simulink model "full_maneuver_platoon"  (R2022a)
settings: Solver=ode23t  StartTime=0.0  StopTime=300  FixedStep=0.1  MaxStep=0.01  RelTol=1e-3
InitFcn:
  | totalVehicles = 7;
  | if exist('vehStatesBus', 'var')==0
  | load vehBuses
  | end
  | if exist('vehErrorsBus', 'var')==0
  | load vehBuses
  | end
libraries: simulink x80, powerlib_meascontrol x16, autolibshared x7, dspsigops x4
(part 7 of 9)

== system full_maneuver_platoon/p1/CACC destination lane/Virtual Vehicle Following/Define Desired Distance ==
  extraSpaceFlag : Inport
  Constant : Constant  Value=h
  Constant1 : Constant  Value=d0
  Constant2 : Constant  Value=hLC
  Constant3 : Constant  Value=d0LC
  Demux : Demux  Outputs=2
  Integrator : Integrator  InitialCondition=[h d0]
  Mux : Mux  Inputs=2
  Mux1 : Mux  Inputs=2
  Saturation1 : Saturate  UpperLimit=hFilterSaturation/2  LowerLimit=-hFilterSaturation
  Sum5 : Sum  Inputs=|+-
  Switch : Switch  Criteria=u2 > Threshold  SaturateOnIntegerOverflow=off  InputSameDT=off
  hFilterGain : Gain  Gain=hFilterGain
  h : Outport
  d0 : Outport  Port=2
  wires:
  Demux/2 -> d0/1
  Demux/1 -> h/1
  Integrator/1 -> Sum5/2, Demux/1
  Saturation1/1 -> Integrator/1
  extraSpaceFlag/1 -> Switch/2
  Constant1/1 -> Mux/2
  Constant3/1 -> Mux1/2
  Switch/1 -> Sum5/1
  Mux1/1 -> Switch/1
  Sum5/1 -> hFilterGain/1
  Constant2/1 -> Mux1/1
  hFilterGain/1 -> Saturation1/1
  Constant/1 -> Mux/1
  Mux/1 -> Switch/3

== system full_maneuver_platoon/p1/CACC destination lane/Virtual Vehicle Following/Min Velocity Control ==
  ev : Inport
  ea : Inport  Port=2
  intergralReset : Inport  Port=3
  Abs : Abs  SaturateOnIntegerOverflow=off
  Compare To Constant : simulink/Logic and Bit Operations/Compare To Constant  relop=<=  const=2*maxComfAccel  OutDataTypeStr=boolean
  Gain : Gain  Gain=velKd
  Scope : Scope  NumInputPorts=4
  Sum3 : Sum  Inputs=+++
  Transport Delay : TransportDelay  DelayTime=0.1
  integral term : Subsystem
  velKp : Gain  Gain=velKp
  u : Outport  VectorParamsAs1DForOutWhenUnconnected=off
  wires:
  Compare To Constant/1 -> integral term/Enable
  integral term/1(Out1) -> Sum3/1, Scope/1
  Abs/1 -> Compare To Constant/1
  Transport Delay/1 -> Abs/1
  ev/1 -> velKp/1, integral term/1(ev)
  velKp/1 -> Scope/2, Sum3/2
  Sum3/1 -> u/1, Scope/4, Transport Delay/1
  intergralReset/1 -> integral term/2(intergralReset)
  ea/1 -> Gain/1
  Gain/1 -> Scope/3, Sum3/3

== system full_maneuver_platoon/p1/CACC destination lane/Virtual Vehicle Following/Velocity Error ==
  ego : Inport
  velRef : Inport  Port=2
  filterReset : Inport  Port=3
  Bus Selector : BusSelector  OutputSignals=Xdot,xddot
  Gain : Gain  Gain=-1
  Gain3 : Gain  Gain=velFilterGain
  Integrator1 : Integrator  ExternalReset=rising  InitialConditionSource=external  InitialCondition=vx0
  Saturation : Saturate  UpperLimit=maxComfAccel  LowerLimit=minComfAccel
  Sum : Sum  Inputs=+-|
  Sum8 : Sum  Inputs=|+-
  ev : Outport
  ea : Outport  Port=2
  wires:
  Sum8/1 -> Gain3/1
  Gain3/1 -> Saturation/1
  Saturation/1 -> Integrator1/1
  velRef/1 -> Sum8/1
  Integrator1/1 -> Sum/1, Sum8/2
  ego/1 -> Bus Selector/1
  Bus Selector/1 -> Sum/2, Integrator1/3  "<Xdot>"
  Bus Selector/2 -> Gain/1  "<xddot>"
  Sum/1 -> ev/1
  Gain/1 -> ea/1
  filterReset/1 -> Integrator1/2

== system full_maneuver_platoon/p1/CACC destination lane/Virtual Vehicle Following/Virtual Leader Following ==
  errors : Inport
  errorsDot : Inport  Port=2
  realInput : Inport  Port=3
  leaderChange : Inport  Port=4
  inRange : Inport  Port=5
  AND : Logic  IconShape=distinctive  AllPortsSameDT=off  OutDataTypeStr=boolean
  Compare To Constant : simulink/Logic and Bit Operations/Compare To Constant  relop=~=  const=0  OutDataTypeStr=boolean
  Constant : Constant  Value=Ki
  Demux : Demux  Outputs=2
  Demux1 : Demux  Outputs=2
  Gain3 : Gain  Gain=Ka
  Gain4 : Gain  Gain=Kdd
  Gain5 : Gain  Commented=on  Gain=10
  Integrator1 : Integrator  Commented=on  ExternalReset=rising  InitialConditionSource=external  InitialCondition=vx0
  Kd : Gain  Gain=Kd
  Kp : Gain  Gain=Kp
  Saturation : Saturate  Commented=on  UpperLimit=maxComfAccel  LowerLimit=minAcceleration
  Saturation1 : Saturate  UpperLimit=maxGapError  LowerLimit=minGapError
  Scope : Scope  NumInputPorts=6
  Sum : Sum  Inputs=+-|
  Sum1 : Sum  Inputs=+++++
  Sum8 : Sum  Commented=on  Inputs=|+-
  Transport Delay : TransportDelay  DelayTime=0.1
  integralTerm : Subsystem
  u : Outport  VectorParamsAs1DForOutWhenUnconnected=off
  wires:
  errorsDot/1 -> Demux1/1
  errors/1 -> Demux/1
  Demux/1 -> Saturation1/1
  Kd/1 -> Scope/3, Sum1/3
  Gain5/1 -> Saturation/1
  inRange/1 -> AND/2, Integrator1/2
  Transport Delay/1 -> Scope/1, Sum1/1
  Saturation1/1 -> integralTerm/1(eh), Kp/1
  Kp/1 -> Scope/2, Sum1/2
  Sum/1 -> integralTerm/2(inputDiff)
  Sum8/1 -> Gain5/1
  realInput/1 -> Integrator1/3, Sum/2
  Gain4/1 -> Scope/4, Sum1/4
  Saturation/1 -> Integrator1/1
  Demux/2 -> Kd/1  "ev"
  Gain3/1 -> Scope/5, Sum1/5
  Integrator1/1 -> Sum8/2
  Sum1/1 -> u/1, Scope/6, Sum/1
  integralTerm/1(Out1) -> Transport Delay/1
  leaderChange/1 -> integralTerm/3(leaderChange)
  Demux1/1 -> Gain4/1  "egDot"
  Demux1/2 -> Gain3/1  "evDot"
  Constant/1 -> Compare To Constant/1
  Compare To Constant/1 -> AND/1
  AND/1 -> integralTerm/Enable

== system full_maneuver_platoon/p1/CACC destination lane/Virtual Vehicle Following/switch min vel ==
  errors : Inport
  errorsDot : Inport  Port=2
  gap : Inport  Port=3
  h : Inport  Port=4
  d0 : Inport  Port=5
  vRef : Inport  Port=6
  Demux1 : Demux  Outputs=2
  Gain1 : Gain
  MATLAB Function : MATLAB Function  TreatAsAtomicUnit=on
  Relay1 : Relay  OnSwitchValue=1  OffSwitchValue=-1
  Scope : Scope  NumInputPorts=2
  Selector : Selector  InputPortWidth=2  IndexOptions=Index vector (dialog)  Indices=[2]  OutputSizes=1
  Sum2 : Sum  Inputs=-+
  inRange : Outport  VectorParamsAs1DForOutWhenUnconnected=off
  wires:
  Demux1/2 -> MATLAB Function/6(ea)
  Demux1/1 -> MATLAB Function/5(ehDot)
  errorsDot/1 -> Demux1/1
  MATLAB Function/1(maxGap) -> Sum2/2, Scope/2
  Gain1/1 -> MATLAB Function/1(h)
  Relay1/1 -> inRange/1
  Selector/1 -> MATLAB Function/4(ev)
  Sum2/1 -> Relay1/1
  gap/1 -> Sum2/1, Scope/1
  errors/1 -> Selector/1
  h/1 -> Gain1/1
  vRef/1 -> MATLAB Function/3(vRef)
  d0/1 -> MATLAB Function/2(d0)

== system full_maneuver_platoon/p1/CACC origin lane/Veh Following/integralTerm ==
  eh : Inport
  inputDiff : Inport  Port=2
  leaderChange : Inport  Port=3
  Enable : EnablePort  ShowOutputPort=on
  Anti-windup gain : Gain  Gain=sqrt(Ki/Kd)
  Integrator : Integrator  ExternalReset=either
  Ki : Gain  Gain=Ki
  Scope : Scope  NumInputPorts=2
  Sum5 : Sum  Inputs=-+|
  XOR : Logic  Operator=XOR  IconShape=distinctive  AllPortsSameDT=off  OutDataTypeStr=boolean
  Out1 : Outport  OutputWhenDisabled=reset  InitialOutput=0  VectorParamsAs1DForOutWhenUnconnected=off
  wires:
  inputDiff/1 -> Anti-windup gain/1
  Anti-windup gain/1 -> Scope/1, Sum5/1
  Ki/1 -> Sum5/2
  Sum5/1 -> Scope/2, Integrator/1
  Enable/1 -> XOR/2
  leaderChange/1 -> XOR/1
  XOR/1 -> Integrator/2
  Integrator/1 -> Out1/1
  eh/1 -> Ki/1

== system full_maneuver_platoon/p1/CACC origin lane/Velocity Control/integral term ==
  ev : Inport
  integralReset : Inport  Port=2
  Enable : EnablePort  StatesWhenEnabling=reset
  Integrator2 : Integrator  ExternalReset=rising
  velKi : Gain  Gain=velKi
  Out1 : Outport  OutputWhenDisabled=reset  InitialOutput=0
  wires:
  ev/1 -> velKi/1
  Integrator2/1 -> Out1/1
  velKi/1 -> Integrator2/1
  integralReset/1 -> Integrator2/2

== system full_maneuver_platoon/p1/Lane Change Strategy/Strategy 1: synchronous/determine virtual follower idx ==
  note: In the synchronous strategy, only the last platoon vehicles has a virtual follower,
      | which is the follower in the destination lane (fd) as virtual follower. The index of
      | fd in the allVehicles array is 2
  Enable : EnablePort
  Constant : Constant  Value=2
  virtualFollowerIdx : Outport  OutputWhenDisabled=reset  InitialOutput=[0]
  wires:
  Constant/1 -> virtualFollowerIdx/1

== system full_maneuver_platoon/p1/Lane Change Strategy/Strategy 1: synchronous/determine virtual leader idx ==
  nVehicles : Inport
  lcFlag : Inport  Port=2
  Enable : EnablePort
  determineVirtualLeader : MATLAB Function  TreatAsAtomicUnit=on
  virtualLeaderIdx : Outport  InitialOutput=0
  wires:
  lcFlag/1 -> determineVirtualLeader/2(lcFlag)
  determineVirtualLeader/1(virtualLeaderIdx) -> virtualLeaderIdx/1
  nVehicles/1 -> determineVirtualLeader/1(nVehicles)

== system full_maneuver_platoon/p1/Lane Change Strategy/Strategy 2: leader first/determine virtual follower idx ==
  note: In the leader first strategy, all vehicles have the follower in the destination lane (fd)
      | as virtual follower. The index of fd in the allVehicles array is 2
  Enable : EnablePort
  Constant : Constant  Value=2
  virtualFollowerIdx : Outport  OutputWhenDisabled=reset  InitialOutput=[0]
  wires:
  Constant/1 -> virtualFollowerIdx/1

== system full_maneuver_platoon/p1/Lane Change Strategy/Strategy 2: leader first/determine virtual leader idx ==
  nVehicles : Inport
  lcFlag : Inport  Port=2
  posInPlatoon : Inport  Port=3
  Enable : EnablePort
  determineVirtualLeader : MATLAB Function  TreatAsAtomicUnit=on
  virtualLeaderIdx : Outport  InitialOutput=[0]
  wires:
  posInPlatoon/1 -> determineVirtualLeader/3(posInPlatoon)
  determineVirtualLeader/1(virtualLeaderIdx) -> virtualLeaderIdx/1  "virtualLeaderIdx"
  lcFlag/1 -> determineVirtualLeader/2(lcFlag)
  nVehicles/1 -> determineVirtualLeader/1(nVehicles)

== system full_maneuver_platoon/p1/Lane Change Strategy/Strategy 3: last first/determine virtual follower idx ==
  platoonSize : Inport
  posInPlatoon : Inport  Port=2
  Enable : EnablePort
  determineVirtualFollower : MATLAB Function  TreatAsAtomicUnit=on
  virtual follower idx : Outport  OutputWhenDisabled=reset  InitialOutput=[0]
  wires:
  posInPlatoon/1 -> determineVirtualFollower/2(posInPlatoon)
  determineVirtualFollower/1(virtualFollowerIdx) -> virtual follower idx/1
  platoonSize/1 -> determineVirtualFollower/1(platoonSize)

== system full_maneuver_platoon/p1/Lane Change Strategy/Strategy 3: last first/determine virtual leader idx ==
  nVehicles : Inport
  lcFlag : Inport  Port=2
  lcDone : Inport  Port=3
  posInPlatoon : Inport  Port=4
  Enable : EnablePort
  determineVirtualLeader : MATLAB Function  TreatAsAtomicUnit=on
  virtualLeaderIdx : Outport  InitialOutput=[0]
  wires:
  nVehicles/1 -> determineVirtualLeader/1(nVehicles)
  posInPlatoon/1 -> determineVirtualLeader/4(posInPlatoon)
  lcFlag/1 -> determineVirtualLeader/2(lcFlag)
  lcDone/1 -> determineVirtualLeader/3(lcDone)
  determineVirtualLeader/1(virtualLeaderIdx) -> virtualLeaderIdx/1

== system full_maneuver_platoon/p1/Lane Change Strategy/Strategy 4: leader first invert/Subsystem ==
  posInPlatoon : Inport
  Enable : EnablePort
  determineVirtualFollower : MATLAB Function  TreatAsAtomicUnit=on
  virtualFollowerIdx : Outport  OutputWhenDisabled=reset  InitialOutput=[0]
  wires:
  determineVirtualFollower/1(virtualFollowerIdx) -> virtualFollowerIdx/1
  posInPlatoon/1 -> determineVirtualFollower/1(posInPlatoon)

== system full_maneuver_platoon/p1/Lane Change Strategy/Strategy 4: leader first invert/Subsystem1 ==
  nVehicles : Inport
  lcFlag : Inport  Port=2
  lcDone : Inport  Port=3
  posInPlatoon : Inport  Port=4
  Enable : EnablePort
  determineVirtualLeader : MATLAB Function  TreatAsAtomicUnit=on
  virtualLeaderIdx : Outport  InitialOutput=[0]
  wires:
  lcDone/1 -> determineVirtualLeader/3(lcDone)
  nVehicles/1 -> determineVirtualLeader/1(nVehicles)
  lcFlag/1 -> determineVirtualLeader/2(lcFlag)
  posInPlatoon/1 -> determineVirtualLeader/4(posInPlatoon)
  determineVirtualLeader/1(virtualLeaderIdx) -> virtualLeaderIdx/1

== system full_maneuver_platoon/p2/CACC destination lane/Virtual Vehicle Following/Compute Errors ==
  ego : Inport
  leader : Inport  Port=2
  h : Inport  Port=3
  d0 : Inport  Port=4
  velFilterReset : Inport  Port=5
  Bus Selector1 : BusSelector  OutputSignals=X,Xdot,xddot
  Bus Selector2 : BusSelector  OutputSignals=X,Xdot,xddot
  Compare To Constant : simulink/Logic and Bit Operations/Compare To Constant  relop=<  const=0  OutDataTypeStr=boolean
  Gain3 : Gain  Gain=velFilterGain
  Integrator1 : Integrator  ExternalReset=rising  InitialCondition=vx0
  Multiply : Product
  Multiply1 : Product
  Mux2 : Mux  Inputs=2
  Mux3 : Mux  Inputs=2
  Product : Product
  Saturation : Saturate  UpperLimit=maxAcceleration  LowerLimit=minAcceleration
  Sum : Sum  Inputs=|-+
  Sum1 : Sum  Inputs=|++
  Sum10 : Sum  Inputs=+-|
  Sum2 : Sum  Inputs=+-|
  Sum3 : Sum  Inputs=|++
  Sum4 : Sum  Inputs=-+|
  Sum6 : Sum  Inputs=|-+
  Sum7 : Sum  Inputs=++|
  Sum8 : Sum  Inputs=|+-
  Sum9 : Sum  Inputs=-+|
  min d0 : Constant  Value=d0
  min h : Constant  Value=h
  vLen : Constant  Value=lr+lf
  errors : Outport  VectorParamsAs1DForOutWhenUnconnected=off
  errorsDot : Outport  Port=2
  "gap " : Outport  Port=3  VectorParamsAs1DForOutWhenUnconnected=off
  unsafeFlag : Outport  Port=4  VectorParamsAs1DForOutWhenUnconnected=off
  wires:
  Mux2/1 -> errors/1
  velFilterReset/1 -> Integrator1/2
  Sum6/1 -> Compare To Constant/1
  Sum7/1 -> Sum6/1  "safe  gap"
  min h/1 -> Product/1
  Compare To Constant/1 -> unsafeFlag/1
  Sum2/1 -> Mux2/1  "eg"
  Bus Selector1/1 -> Sum/2  "<X>"
  Product/1 -> Sum7/2
  Sum3/1 -> Sum2/2  "desired  gap"
  Sum1/1 -> Sum/1  "x (front bumber)"
  Bus Selector2/2 -> Sum4/1, Multiply/1, Product/2  "<Xdot>"
  d0/1 -> Sum3/2
  vLen/1 -> Sum1/1
  min d0/1 -> Sum7/1
  Multiply/1 -> Sum3/1
  Sum/1 -> Sum2/1, "gap "/1, Sum6/2  "gap"
  Bus Selector2/1 -> Sum1/2  "<X>"
  h/1 -> Multiply/2, Multiply1/1
  Bus Selector1/2 -> Sum8/1  "<Xdot>"
  Sum4/1 -> Mux2/2, Sum10/1  "ev"
  Gain3/1 -> Saturation/1
  Saturation/1 -> Integrator1/1
  Integrator1/1 -> Sum4/2, Sum8/2
  Sum8/1 -> Gain3/1
  Bus Selector1/3 -> Sum9/2  "<xddot>"
  Bus Selector2/3 -> Sum9/1, Multiply1/2  "<xddot>"
  Multiply1/1 -> Sum10/2
  Sum10/1 -> Mux3/1  "egDot"
  Sum9/1 -> Mux3/2  "evDot"
  Mux3/1 -> errorsDot/1
  ego/1 -> Bus Selector2/1
  leader/1 -> Bus Selector1/1

== system full_maneuver_platoon/p2/CACC destination lane/Virtual Vehicle Following/Define Desired Distance ==
  extraSpaceFlag : Inport
  Constant : Constant  Value=h
  Constant1 : Constant  Value=d0
  Constant2 : Constant  Value=hLC
  Constant3 : Constant  Value=d0LC
  Demux : Demux  Outputs=2
  Integrator : Integrator  InitialCondition=[h d0]
  Mux : Mux  Inputs=2
  Mux1 : Mux  Inputs=2
  Saturation1 : Saturate  UpperLimit=hFilterSaturation/2  LowerLimit=-hFilterSaturation
  Sum5 : Sum  Inputs=|+-
  Switch : Switch  Criteria=u2 > Threshold  SaturateOnIntegerOverflow=off  InputSameDT=off
  hFilterGain : Gain  Gain=hFilterGain
  h : Outport
  d0 : Outport  Port=2
  wires:
  Mux/1 -> Switch/3
  Constant/1 -> Mux/1
  hFilterGain/1 -> Saturation1/1
  Constant2/1 -> Mux1/1
  Sum5/1 -> hFilterGain/1
  Mux1/1 -> Switch/1
  Switch/1 -> Sum5/1
  Constant3/1 -> Mux1/2
  Constant1/1 -> Mux/2
  extraSpaceFlag/1 -> Switch/2
  Saturation1/1 -> Integrator/1
  Integrator/1 -> Demux/1, Sum5/2
  Demux/1 -> h/1
  Demux/2 -> d0/1

== system full_maneuver_platoon/p2/CACC destination lane/Virtual Vehicle Following/Min Velocity Control ==
  ev : Inport
  ea : Inport  Port=2
  intergralReset : Inport  Port=3
  Abs : Abs  SaturateOnIntegerOverflow=off
  Compare To Constant : simulink/Logic and Bit Operations/Compare To Constant  relop=<=  const=2*maxComfAccel  OutDataTypeStr=boolean
  Gain : Gain  Gain=velKd
  Scope : Scope  NumInputPorts=4
  Sum3 : Sum  Inputs=+++
  Transport Delay : TransportDelay  DelayTime=0.1
  integral term : Subsystem
  velKp : Gain  Gain=velKp
  u : Outport  VectorParamsAs1DForOutWhenUnconnected=off
  wires:
  Gain/1 -> Sum3/3, Scope/3
  ea/1 -> Gain/1
  intergralReset/1 -> integral term/2(intergralReset)
  Sum3/1 -> Transport Delay/1, Scope/4, u/1
  velKp/1 -> Sum3/2, Scope/2
  ev/1 -> integral term/1(ev), velKp/1
  Transport Delay/1 -> Abs/1
  Abs/1 -> Compare To Constant/1
  integral term/1(Out1) -> Scope/1, Sum3/1
  Compare To Constant/1 -> integral term/Enable

== system full_maneuver_platoon/p2/CACC destination lane/Virtual Vehicle Following/Velocity Error ==
  ego : Inport
  velRef : Inport  Port=2
  filterReset : Inport  Port=3
  Bus Selector : BusSelector  OutputSignals=Xdot,xddot
  Gain : Gain  Gain=-1
  Gain3 : Gain  Gain=velFilterGain
  Integrator1 : Integrator  ExternalReset=rising  InitialConditionSource=external  InitialCondition=vx0
  Saturation : Saturate  UpperLimit=maxComfAccel  LowerLimit=minComfAccel
  Sum : Sum  Inputs=+-|
  Sum8 : Sum  Inputs=|+-
  ev : Outport
  ea : Outport  Port=2
  wires:
  filterReset/1 -> Integrator1/2
  Gain/1 -> ea/1
  Sum/1 -> ev/1
  Bus Selector/2 -> Gain/1  "<xddot>"
  Bus Selector/1 -> Integrator1/3, Sum/2  "<Xdot>"
  ego/1 -> Bus Selector/1
  Integrator1/1 -> Sum8/2, Sum/1
  velRef/1 -> Sum8/1
  Saturation/1 -> Integrator1/1
  Gain3/1 -> Saturation/1
  Sum8/1 -> Gain3/1

== system full_maneuver_platoon/p2/CACC destination lane/Virtual Vehicle Following/Virtual Leader Following ==
  errors : Inport
  errorsDot : Inport  Port=2
  realInput : Inport  Port=3
  leaderChange : Inport  Port=4
  inRange : Inport  Port=5
  AND : Logic  IconShape=distinctive  AllPortsSameDT=off  OutDataTypeStr=boolean
  Compare To Constant : simulink/Logic and Bit Operations/Compare To Constant  relop=~=  const=0  OutDataTypeStr=boolean
  Constant : Constant  Value=Ki
  Demux : Demux  Outputs=2
  Demux1 : Demux  Outputs=2
  Gain3 : Gain  Gain=Ka
  Gain4 : Gain  Gain=Kdd
  Gain5 : Gain  Commented=on  Gain=10
  Integrator1 : Integrator  Commented=on  ExternalReset=rising  InitialConditionSource=external  InitialCondition=vx0
  Kd : Gain  Gain=Kd
  Kp : Gain  Gain=Kp
  Saturation : Saturate  Commented=on  UpperLimit=maxComfAccel  LowerLimit=minAcceleration
  Saturation1 : Saturate  UpperLimit=maxGapError  LowerLimit=minGapError
  Scope : Scope  NumInputPorts=6
  Sum : Sum  Inputs=+-|
  Sum1 : Sum  Inputs=+++++
  Sum8 : Sum  Commented=on  Inputs=|+-
  Transport Delay : TransportDelay  DelayTime=0.1
  integralTerm : Subsystem
  u : Outport  VectorParamsAs1DForOutWhenUnconnected=off
  wires:
  AND/1 -> integralTerm/Enable
  Compare To Constant/1 -> AND/1
  Constant/1 -> Compare To Constant/1
  Demux1/2 -> Gain3/1  "evDot"
  Demux1/1 -> Gain4/1  "egDot"
  leaderChange/1 -> integralTerm/3(leaderChange)
  integralTerm/1(Out1) -> Transport Delay/1
  Sum1/1 -> Sum/1, Scope/6, u/1
  Integrator1/1 -> Sum8/2
  Gain3/1 -> Sum1/5, Scope/5
  Demux/2 -> Kd/1  "ev"
  Saturation/1 -> Integrator1/1
  Gain4/1 -> Sum1/4, Scope/4
  realInput/1 -> Sum/2, Integrator1/3
  Sum8/1 -> Gain5/1
  Sum/1 -> integralTerm/2(inputDiff)
  Kp/1 -> Sum1/2, Scope/2
  Saturation1/1 -> Kp/1, integralTerm/1(eh)
  Transport Delay/1 -> Sum1/1, Scope/1
  inRange/1 -> Integrator1/2, AND/2
  Gain5/1 -> Saturation/1
  Kd/1 -> Sum1/3, Scope/3
  Demux/1 -> Saturation1/1
  errors/1 -> Demux/1
  errorsDot/1 -> Demux1/1

== system full_maneuver_platoon/p2/CACC destination lane/Virtual Vehicle Following/switch min vel ==
  errors : Inport
  errorsDot : Inport  Port=2
  gap : Inport  Port=3
  h : Inport  Port=4
  d0 : Inport  Port=5
  vRef : Inport  Port=6
  Demux1 : Demux  Outputs=2
  Gain1 : Gain
  MATLAB Function : MATLAB Function  TreatAsAtomicUnit=on
  Relay1 : Relay  OnSwitchValue=1  OffSwitchValue=-1
  Scope : Scope  NumInputPorts=2
  Selector : Selector  InputPortWidth=2  IndexOptions=Index vector (dialog)  Indices=[2]  OutputSizes=1
  Sum2 : Sum  Inputs=-+
  inRange : Outport  VectorParamsAs1DForOutWhenUnconnected=off
  wires:
  d0/1 -> MATLAB Function/2(d0)
  vRef/1 -> MATLAB Function/3(vRef)
  h/1 -> Gain1/1
  errors/1 -> Selector/1
  gap/1 -> Scope/1, Sum2/1
  Sum2/1 -> Relay1/1
  Selector/1 -> MATLAB Function/4(ev)
  Relay1/1 -> inRange/1
  Gain1/1 -> MATLAB Function/1(h)
  MATLAB Function/1(maxGap) -> Scope/2, Sum2/2
  errorsDot/1 -> Demux1/1
  Demux1/1 -> MATLAB Function/5(ehDot)
  Demux1/2 -> MATLAB Function/6(ea)

== system full_maneuver_platoon/p2/CACC origin lane/Veh Following/integralTerm ==
  eh : Inport
  inputDiff : Inport  Port=2
  leaderChange : Inport  Port=3
  Enable : EnablePort  ShowOutputPort=on
  Anti-windup gain : Gain  Gain=sqrt(Ki/Kd)
  Integrator : Integrator  ExternalReset=either
  Ki : Gain  Gain=Ki
  Scope : Scope  NumInputPorts=2
  Sum5 : Sum  Inputs=-+|
  XOR : Logic  Operator=XOR  IconShape=distinctive  AllPortsSameDT=off  OutDataTypeStr=boolean
  Out1 : Outport  OutputWhenDisabled=reset  InitialOutput=0  VectorParamsAs1DForOutWhenUnconnected=off
  wires:
  eh/1 -> Ki/1
  Integrator/1 -> Out1/1
  XOR/1 -> Integrator/2
  leaderChange/1 -> XOR/1
  Enable/1 -> XOR/2
  Sum5/1 -> Integrator/1, Scope/2
  Ki/1 -> Sum5/2
  Anti-windup gain/1 -> Sum5/1, Scope/1
  inputDiff/1 -> Anti-windup gain/1

== system full_maneuver_platoon/p2/CACC origin lane/Velocity Control/integral term ==
  ev : Inport
  integralReset : Inport  Port=2
  Enable : EnablePort  StatesWhenEnabling=reset
  Integrator2 : Integrator  ExternalReset=rising
  velKi : Gain  Gain=velKi
  Out1 : Outport  OutputWhenDisabled=reset  InitialOutput=0
  wires:
  integralReset/1 -> Integrator2/2
  velKi/1 -> Integrator2/1
  Integrator2/1 -> Out1/1
  ev/1 -> velKi/1

== system full_maneuver_platoon/p2/Lane Change Strategy/Strategy 1: synchronous/determine virtual follower idx ==
  note: In the synchronous strategy, only the last platoon vehicles has a virtual follower,
      | which is the follower in the destination lane (fd) as virtual follower. The index of
      | fd in the allVehicles array is 2
  Enable : EnablePort
  Constant : Constant  Value=2
  virtualFollowerIdx : Outport  OutputWhenDisabled=reset  InitialOutput=[0]
  wires:
  Constant/1 -> virtualFollowerIdx/1

== system full_maneuver_platoon/p2/Lane Change Strategy/Strategy 1: synchronous/determine virtual leader idx ==
  nVehicles : Inport
  lcFlag : Inport  Port=2
  Enable : EnablePort
  determineVirtualLeader : MATLAB Function  TreatAsAtomicUnit=on
  virtualLeaderIdx : Outport  InitialOutput=0
  wires:
  nVehicles/1 -> determineVirtualLeader/1(nVehicles)
  determineVirtualLeader/1(virtualLeaderIdx) -> virtualLeaderIdx/1
  lcFlag/1 -> determineVirtualLeader/2(lcFlag)

== system full_maneuver_platoon/p2/Lane Change Strategy/Strategy 2: leader first/determine virtual follower idx ==
  note: In the leader first strategy, all vehicles have the follower in the destination lane (fd)
      | as virtual follower. The index of fd in the allVehicles array is 2
  Enable : EnablePort
  Constant : Constant  Value=2
  virtualFollowerIdx : Outport  OutputWhenDisabled=reset  InitialOutput=[0]
  wires:
  Constant/1 -> virtualFollowerIdx/1

== system full_maneuver_platoon/p2/Lane Change Strategy/Strategy 2: leader first/determine virtual leader idx ==
  nVehicles : Inport
  lcFlag : Inport  Port=2
  posInPlatoon : Inport  Port=3
  Enable : EnablePort
  determineVirtualLeader : MATLAB Function  TreatAsAtomicUnit=on
  virtualLeaderIdx : Outport  InitialOutput=[0]
  wires:
  nVehicles/1 -> determineVirtualLeader/1(nVehicles)
  lcFlag/1 -> determineVirtualLeader/2(lcFlag)
  determineVirtualLeader/1(virtualLeaderIdx) -> virtualLeaderIdx/1  "virtualLeaderIdx"
  posInPlatoon/1 -> determineVirtualLeader/3(posInPlatoon)

== system full_maneuver_platoon/p2/Lane Change Strategy/Strategy 3: last first/determine virtual follower idx ==
  platoonSize : Inport
  posInPlatoon : Inport  Port=2
  Enable : EnablePort
  determineVirtualFollower : MATLAB Function  TreatAsAtomicUnit=on
  virtual follower idx : Outport  OutputWhenDisabled=reset  InitialOutput=[0]
  wires:
  platoonSize/1 -> determineVirtualFollower/1(platoonSize)
  determineVirtualFollower/1(virtualFollowerIdx) -> virtual follower idx/1
  posInPlatoon/1 -> determineVirtualFollower/2(posInPlatoon)

== system full_maneuver_platoon/p2/Lane Change Strategy/Strategy 3: last first/determine virtual leader idx ==
  nVehicles : Inport
  lcFlag : Inport  Port=2
  lcDone : Inport  Port=3
  posInPlatoon : Inport  Port=4
  Enable : EnablePort
  determineVirtualLeader : MATLAB Function  TreatAsAtomicUnit=on
  virtualLeaderIdx : Outport  InitialOutput=[0]
  wires:
  determineVirtualLeader/1(virtualLeaderIdx) -> virtualLeaderIdx/1
  lcDone/1 -> determineVirtualLeader/3(lcDone)
  lcFlag/1 -> determineVirtualLeader/2(lcFlag)
  posInPlatoon/1 -> determineVirtualLeader/4(posInPlatoon)
  nVehicles/1 -> determineVirtualLeader/1(nVehicles)

== system full_maneuver_platoon/p2/Lane Change Strategy/Strategy 4: leader first invert/Subsystem ==
  posInPlatoon : Inport
  Enable : EnablePort
  determineVirtualFollower : MATLAB Function  TreatAsAtomicUnit=on
  virtualFollowerIdx : Outport  OutputWhenDisabled=reset  InitialOutput=[0]
  wires:
  posInPlatoon/1 -> determineVirtualFollower/1(posInPlatoon)
  determineVirtualFollower/1(virtualFollowerIdx) -> virtualFollowerIdx/1

== system full_maneuver_platoon/p2/Lane Change Strategy/Strategy 4: leader first invert/Subsystem1 ==
  nVehicles : Inport
  lcFlag : Inport  Port=2
  lcDone : Inport  Port=3
  posInPlatoon : Inport  Port=4
  Enable : EnablePort
  determineVirtualLeader : MATLAB Function  TreatAsAtomicUnit=on
  virtualLeaderIdx : Outport  InitialOutput=[0]
  wires:
  determineVirtualLeader/1(virtualLeaderIdx) -> virtualLeaderIdx/1
  posInPlatoon/1 -> determineVirtualLeader/4(posInPlatoon)
  lcFlag/1 -> determineVirtualLeader/2(lcFlag)
  nVehicles/1 -> determineVirtualLeader/1(nVehicles)
  lcDone/1 -> determineVirtualLeader/3(lcDone)

== system full_maneuver_platoon/p3/CACC destination lane/Virtual Vehicle Following/Compute Errors ==
  ego : Inport
  leader : Inport  Port=2
  h : Inport  Port=3
  d0 : Inport  Port=4
  velFilterReset : Inport  Port=5
  Bus Selector1 : BusSelector  OutputSignals=X,Xdot,xddot
  Bus Selector2 : BusSelector  OutputSignals=X,Xdot,xddot
  Compare To Constant : simulink/Logic and Bit Operations/Compare To Constant  relop=<  const=0  OutDataTypeStr=boolean
  Gain3 : Gain  Gain=velFilterGain
  Integrator1 : Integrator  ExternalReset=rising  InitialCondition=vx0
  Multiply : Product
  Multiply1 : Product
  Mux2 : Mux  Inputs=2
  Mux3 : Mux  Inputs=2
  Product : Product
  Saturation : Saturate  UpperLimit=maxAcceleration  LowerLimit=minAcceleration
  Sum : Sum  Inputs=|-+
  Sum1 : Sum  Inputs=|++
  Sum10 : Sum  Inputs=+-|
  Sum2 : Sum  Inputs=+-|
  Sum3 : Sum  Inputs=|++
  Sum4 : Sum  Inputs=-+|
  Sum6 : Sum  Inputs=|-+
  Sum7 : Sum  Inputs=++|
  Sum8 : Sum  Inputs=|+-
  Sum9 : Sum  Inputs=-+|
  min d0 : Constant  Value=d0
  min h : Constant  Value=h
  vLen : Constant  Value=lr+lf
  errors : Outport  VectorParamsAs1DForOutWhenUnconnected=off
  errorsDot : Outport  Port=2
  "gap " : Outport  Port=3  VectorParamsAs1DForOutWhenUnconnected=off
  unsafeFlag : Outport  Port=4  VectorParamsAs1DForOutWhenUnconnected=off
  wires:
  leader/1 -> Bus Selector1/1
  ego/1 -> Bus Selector2/1
  Mux3/1 -> errorsDot/1
  Sum9/1 -> Mux3/2  "evDot"
  Sum10/1 -> Mux3/1  "egDot"
  Multiply1/1 -> Sum10/2
  Bus Selector2/3 -> Multiply1/2, Sum9/1  "<xddot>"
  Bus Selector1/3 -> Sum9/2  "<xddot>"
  Sum8/1 -> Gain3/1
  Integrator1/1 -> Sum8/2, Sum4/2
  Saturation/1 -> Integrator1/1
  Gain3/1 -> Saturation/1
  Sum4/1 -> Sum10/1, Mux2/2  "ev"
  Bus Selector1/2 -> Sum8/1  "<Xdot>"
  h/1 -> Multiply1/1, Multiply/2
  Bus Selector2/1 -> Sum1/2  "<X>"
  Sum/1 -> Sum6/2, "gap "/1, Sum2/1  "gap"
  Multiply/1 -> Sum3/1
  min d0/1 -> Sum7/1
  vLen/1 -> Sum1/1
  d0/1 -> Sum3/2
  Bus Selector2/2 -> Product/2, Multiply/1, Sum4/1  "<Xdot>"
  Sum1/1 -> Sum/1  "x (front bumber)"
  Sum3/1 -> Sum2/2  "desired  gap"
  Product/1 -> Sum7/2
  Bus Selector1/1 -> Sum/2  "<X>"
  Sum2/1 -> Mux2/1  "eg"
  Compare To Constant/1 -> unsafeFlag/1
  min h/1 -> Product/1
  Sum7/1 -> Sum6/1  "safe  gap"
  Sum6/1 -> Compare To Constant/1
  velFilterReset/1 -> Integrator1/2
  Mux2/1 -> errors/1

== system full_maneuver_platoon/p3/CACC destination lane/Virtual Vehicle Following/Define Desired Distance ==
  extraSpaceFlag : Inport
  Constant : Constant  Value=h
  Constant1 : Constant  Value=d0
  Constant2 : Constant  Value=hLC
  Constant3 : Constant  Value=d0LC
  Demux : Demux  Outputs=2
  Integrator : Integrator  InitialCondition=[h d0]
  Mux : Mux  Inputs=2
  Mux1 : Mux  Inputs=2
  Saturation1 : Saturate  UpperLimit=hFilterSaturation/2  LowerLimit=-hFilterSaturation
  Sum5 : Sum  Inputs=|+-
  Switch : Switch  Criteria=u2 > Threshold  SaturateOnIntegerOverflow=off  InputSameDT=off
  hFilterGain : Gain  Gain=hFilterGain
  h : Outport
  d0 : Outport  Port=2
  wires:
  Demux/2 -> d0/1
  Demux/1 -> h/1
  Integrator/1 -> Sum5/2, Demux/1
  Saturation1/1 -> Integrator/1
  extraSpaceFlag/1 -> Switch/2
  Constant1/1 -> Mux/2
  Constant3/1 -> Mux1/2
  Switch/1 -> Sum5/1
  Mux1/1 -> Switch/1
  Sum5/1 -> hFilterGain/1
  Constant2/1 -> Mux1/1
  hFilterGain/1 -> Saturation1/1
  Constant/1 -> Mux/1
  Mux/1 -> Switch/3

== system full_maneuver_platoon/p3/CACC destination lane/Virtual Vehicle Following/Min Velocity Control ==
  ev : Inport
  ea : Inport  Port=2
  intergralReset : Inport  Port=3
  Abs : Abs  SaturateOnIntegerOverflow=off
  Compare To Constant : simulink/Logic and Bit Operations/Compare To Constant  relop=<=  const=2*maxComfAccel  OutDataTypeStr=boolean
  Gain : Gain  Gain=velKd
  Scope : Scope  NumInputPorts=4
  Sum3 : Sum  Inputs=+++
  Transport Delay : TransportDelay  DelayTime=0.1
  integral term : Subsystem
  velKp : Gain  Gain=velKp
  u : Outport  VectorParamsAs1DForOutWhenUnconnected=off
  wires:
  Compare To Constant/1 -> integral term/Enable
  integral term/1(Out1) -> Sum3/1, Scope/1
  Abs/1 -> Compare To Constant/1
  Transport Delay/1 -> Abs/1
  ev/1 -> velKp/1, integral term/1(ev)
  velKp/1 -> Scope/2, Sum3/2
  Sum3/1 -> u/1, Scope/4, Transport Delay/1
  intergralReset/1 -> integral term/2(intergralReset)
  ea/1 -> Gain/1
  Gain/1 -> Scope/3, Sum3/3

== system full_maneuver_platoon/p3/CACC destination lane/Virtual Vehicle Following/Velocity Error ==
  ego : Inport
  velRef : Inport  Port=2
  filterReset : Inport  Port=3
  Bus Selector : BusSelector  OutputSignals=Xdot,xddot
  Gain : Gain  Gain=-1
  Gain3 : Gain  Gain=velFilterGain
  Integrator1 : Integrator  ExternalReset=rising  InitialConditionSource=external  InitialCondition=vx0
  Saturation : Saturate  UpperLimit=maxComfAccel  LowerLimit=minComfAccel
  Sum : Sum  Inputs=+-|
  Sum8 : Sum  Inputs=|+-
  ev : Outport
  ea : Outport  Port=2
  wires:
  Sum8/1 -> Gain3/1
  Gain3/1 -> Saturation/1
  Saturation/1 -> Integrator1/1
  velRef/1 -> Sum8/1
  Integrator1/1 -> Sum/1, Sum8/2
  ego/1 -> Bus Selector/1
  Bus Selector/1 -> Sum/2, Integrator1/3  "<Xdot>"
  Bus Selector/2 -> Gain/1  "<xddot>"
  Sum/1 -> ev/1
  Gain/1 -> ea/1
  filterReset/1 -> Integrator1/2

== system full_maneuver_platoon/p3/CACC destination lane/Virtual Vehicle Following/Virtual Leader Following ==
  errors : Inport
  errorsDot : Inport  Port=2
  realInput : Inport  Port=3
  leaderChange : Inport  Port=4
  inRange : Inport  Port=5
  AND : Logic  IconShape=distinctive  AllPortsSameDT=off  OutDataTypeStr=boolean
  Compare To Constant : simulink/Logic and Bit Operations/Compare To Constant  relop=~=  const=0  OutDataTypeStr=boolean
  Constant : Constant  Value=Ki
  Demux : Demux  Outputs=2
  Demux1 : Demux  Outputs=2
  Gain3 : Gain  Gain=Ka
  Gain4 : Gain  Gain=Kdd
  Gain5 : Gain  Commented=on  Gain=10
  Integrator1 : Integrator  Commented=on  ExternalReset=rising  InitialConditionSource=external  InitialCondition=vx0
  Kd : Gain  Gain=Kd
  Kp : Gain  Gain=Kp
  Saturation : Saturate  Commented=on  UpperLimit=maxComfAccel  LowerLimit=minAcceleration
  Saturation1 : Saturate  UpperLimit=maxGapError  LowerLimit=minGapError
  Scope : Scope  NumInputPorts=6
  Sum : Sum  Inputs=+-|
  Sum1 : Sum  Inputs=+++++
  Sum8 : Sum  Commented=on  Inputs=|+-
  Transport Delay : TransportDelay  DelayTime=0.1
  integralTerm : Subsystem
  u : Outport  VectorParamsAs1DForOutWhenUnconnected=off
  wires:
  errorsDot/1 -> Demux1/1
  errors/1 -> Demux/1
  Demux/1 -> Saturation1/1
  Kd/1 -> Scope/3, Sum1/3
  Gain5/1 -> Saturation/1
  inRange/1 -> AND/2, Integrator1/2
  Transport Delay/1 -> Scope/1, Sum1/1
  Saturation1/1 -> integralTerm/1(eh), Kp/1
  Kp/1 -> Scope/2, Sum1/2
  Sum/1 -> integralTerm/2(inputDiff)
  Sum8/1 -> Gain5/1
  realInput/1 -> Integrator1/3, Sum/2
  Gain4/1 -> Scope/4, Sum1/4
  Saturation/1 -> Integrator1/1
  Demux/2 -> Kd/1  "ev"
  Gain3/1 -> Scope/5, Sum1/5
  Integrator1/1 -> Sum8/2
  Sum1/1 -> u/1, Scope/6, Sum/1
  integralTerm/1(Out1) -> Transport Delay/1
  leaderChange/1 -> integralTerm/3(leaderChange)
  Demux1/1 -> Gain4/1  "egDot"
  Demux1/2 -> Gain3/1  "evDot"
  Constant/1 -> Compare To Constant/1
  Compare To Constant/1 -> AND/1
  AND/1 -> integralTerm/Enable

== system full_maneuver_platoon/p3/CACC destination lane/Virtual Vehicle Following/switch min vel ==
  errors : Inport
  errorsDot : Inport  Port=2
  gap : Inport  Port=3
  h : Inport  Port=4
  d0 : Inport  Port=5
  vRef : Inport  Port=6
  Demux1 : Demux  Outputs=2
  Gain1 : Gain
  MATLAB Function : MATLAB Function  TreatAsAtomicUnit=on
  Relay1 : Relay  OnSwitchValue=1  OffSwitchValue=-1
  Scope : Scope  NumInputPorts=2
  Selector : Selector  InputPortWidth=2  IndexOptions=Index vector (dialog)  Indices=[2]  OutputSizes=1
  Sum2 : Sum  Inputs=-+
  inRange : Outport  VectorParamsAs1DForOutWhenUnconnected=off
  wires:
  Demux1/2 -> MATLAB Function/6(ea)
  Demux1/1 -> MATLAB Function/5(ehDot)
  errorsDot/1 -> Demux1/1
  MATLAB Function/1(maxGap) -> Sum2/2, Scope/2
  Gain1/1 -> MATLAB Function/1(h)
  Relay1/1 -> inRange/1
  Selector/1 -> MATLAB Function/4(ev)
  Sum2/1 -> Relay1/1
  gap/1 -> Sum2/1, Scope/1
  errors/1 -> Selector/1
  h/1 -> Gain1/1
  vRef/1 -> MATLAB Function/3(vRef)
  d0/1 -> MATLAB Function/2(d0)

== system full_maneuver_platoon/p3/CACC origin lane/Veh Following/integralTerm ==
  eh : Inport
  inputDiff : Inport  Port=2
  leaderChange : Inport  Port=3
  Enable : EnablePort  ShowOutputPort=on
  Anti-windup gain : Gain  Gain=sqrt(Ki/Kd)
  Integrator : Integrator  ExternalReset=either
  Ki : Gain  Gain=Ki
  Scope : Scope  NumInputPorts=2
  Sum5 : Sum  Inputs=-+|
  XOR : Logic  Operator=XOR  IconShape=distinctive  AllPortsSameDT=off  OutDataTypeStr=boolean
  Out1 : Outport  OutputWhenDisabled=reset  InitialOutput=0  VectorParamsAs1DForOutWhenUnconnected=off
  wires:
  inputDiff/1 -> Anti-windup gain/1
  Anti-windup gain/1 -> Scope/1, Sum5/1
  Ki/1 -> Sum5/2
  Sum5/1 -> Scope/2, Integrator/1
  Enable/1 -> XOR/2
  leaderChange/1 -> XOR/1
  XOR/1 -> Integrator/2
  Integrator/1 -> Out1/1
  eh/1 -> Ki/1

== system full_maneuver_platoon/p3/CACC origin lane/Velocity Control/integral term ==
  ev : Inport
  integralReset : Inport  Port=2
  Enable : EnablePort  StatesWhenEnabling=reset
  Integrator2 : Integrator  ExternalReset=rising
  velKi : Gain  Gain=velKi
  Out1 : Outport  OutputWhenDisabled=reset  InitialOutput=0
  wires:
  ev/1 -> velKi/1
  Integrator2/1 -> Out1/1
  velKi/1 -> Integrator2/1
  integralReset/1 -> Integrator2/2

== system full_maneuver_platoon/p3/Lane Change Strategy/Strategy 1: synchronous/determine virtual follower idx ==
  note: In the synchronous strategy, only the last platoon vehicles has a virtual follower,
      | which is the follower in the destination lane (fd) as virtual follower. The index of
      | fd in the allVehicles array is 2
  Enable : EnablePort
  Constant : Constant  Value=2
  virtualFollowerIdx : Outport  OutputWhenDisabled=reset  InitialOutput=[0]
  wires:
  Constant/1 -> virtualFollowerIdx/1

== system full_maneuver_platoon/p3/Lane Change Strategy/Strategy 1: synchronous/determine virtual leader idx ==
  nVehicles : Inport
  lcFlag : Inport  Port=2
  Enable : EnablePort
  determineVirtualLeader : MATLAB Function  TreatAsAtomicUnit=on
  virtualLeaderIdx : Outport  InitialOutput=0
  wires:
  lcFlag/1 -> determineVirtualLeader/2(lcFlag)
  determineVirtualLeader/1(virtualLeaderIdx) -> virtualLeaderIdx/1
  nVehicles/1 -> determineVirtualLeader/1(nVehicles)

== system full_maneuver_platoon/p3/Lane Change Strategy/Strategy 2: leader first/determine virtual follower idx ==
  note: In the leader first strategy, all vehicles have the follower in the destination lane (fd)
      | as virtual follower. The index of fd in the allVehicles array is 2
  Enable : EnablePort
  Constant : Constant  Value=2
  virtualFollowerIdx : Outport  OutputWhenDisabled=reset  InitialOutput=[0]
  wires:
  Constant/1 -> virtualFollowerIdx/1

== system full_maneuver_platoon/p3/Lane Change Strategy/Strategy 2: leader first/determine virtual leader idx ==
  nVehicles : Inport
  lcFlag : Inport  Port=2
  posInPlatoon : Inport  Port=3
  Enable : EnablePort
  determineVirtualLeader : MATLAB Function  TreatAsAtomicUnit=on
  virtualLeaderIdx : Outport  InitialOutput=[0]
  wires:
  posInPlatoon/1 -> determineVirtualLeader/3(posInPlatoon)
  determineVirtualLeader/1(virtualLeaderIdx) -> virtualLeaderIdx/1  "virtualLeaderIdx"
  lcFlag/1 -> determineVirtualLeader/2(lcFlag)
  nVehicles/1 -> determineVirtualLeader/1(nVehicles)

== system full_maneuver_platoon/p3/Lane Change Strategy/Strategy 3: last first/determine virtual follower idx ==
  platoonSize : Inport
  posInPlatoon : Inport  Port=2
  Enable : EnablePort
  determineVirtualFollower : MATLAB Function  TreatAsAtomicUnit=on
  virtual follower idx : Outport  OutputWhenDisabled=reset  InitialOutput=[0]
  wires:
  posInPlatoon/1 -> determineVirtualFollower/2(posInPlatoon)
  determineVirtualFollower/1(virtualFollowerIdx) -> virtual follower idx/1
  platoonSize/1 -> determineVirtualFollower/1(platoonSize)

== system full_maneuver_platoon/p3/Lane Change Strategy/Strategy 3: last first/determine virtual leader idx ==
  nVehicles : Inport
  lcFlag : Inport  Port=2
  lcDone : Inport  Port=3
  posInPlatoon : Inport  Port=4
  Enable : EnablePort
  determineVirtualLeader : MATLAB Function  TreatAsAtomicUnit=on
  virtualLeaderIdx : Outport  InitialOutput=[0]
  wires:
  nVehicles/1 -> determineVirtualLeader/1(nVehicles)
  posInPlatoon/1 -> determineVirtualLeader/4(posInPlatoon)
  lcFlag/1 -> determineVirtualLeader/2(lcFlag)
  lcDone/1 -> determineVirtualLeader/3(lcDone)
  determineVirtualLeader/1(virtualLeaderIdx) -> virtualLeaderIdx/1

== system full_maneuver_platoon/p3/Lane Change Strategy/Strategy 4: leader first invert/Subsystem ==
  posInPlatoon : Inport
  Enable : EnablePort
  determineVirtualFollower : MATLAB Function  TreatAsAtomicUnit=on
  virtualFollowerIdx : Outport  OutputWhenDisabled=reset  InitialOutput=[0]
  wires:
  determineVirtualFollower/1(virtualFollowerIdx) -> virtualFollowerIdx/1
  posInPlatoon/1 -> determineVirtualFollower/1(posInPlatoon)

== system full_maneuver_platoon/p3/Lane Change Strategy/Strategy 4: leader first invert/Subsystem1 ==
  nVehicles : Inport
  lcFlag : Inport  Port=2
  lcDone : Inport  Port=3
  posInPlatoon : Inport  Port=4
  Enable : EnablePort
  determineVirtualLeader : MATLAB Function  TreatAsAtomicUnit=on
  virtualLeaderIdx : Outport  InitialOutput=[0]
  wires:
  lcDone/1 -> determineVirtualLeader/3(lcDone)
  nVehicles/1 -> determineVirtualLeader/1(nVehicles)
  lcFlag/1 -> determineVirtualLeader/2(lcFlag)
  posInPlatoon/1 -> determineVirtualLeader/4(posInPlatoon)
  determineVirtualLeader/1(virtualLeaderIdx) -> virtualLeaderIdx/1

== system full_maneuver_platoon/Fd/CACC destination lane/Virtual Vehicle Following/Min Velocity Control/integral term ==
  ev : Inport
  intergralReset : Inport  Port=2
  Enable : EnablePort  StatesWhenEnabling=reset
  Integrator2 : Integrator  ExternalReset=rising
  velKi : Gain  Gain=velKi
  Out1 : Outport  OutputWhenDisabled=reset  InitialOutput=0
  wires:
  intergralReset/1 -> Integrator2/2
  velKi/1 -> Integrator2/1
  Integrator2/1 -> Out1/1
  ev/1 -> velKi/1

== system full_maneuver_platoon/Fd/CACC destination lane/Virtual Vehicle Following/Virtual Leader Following/integralTerm ==
  eh : Inport
  inputDiff : Inport  Port=2
  leaderChange : Inport  Port=3
  Enable : EnablePort  ShowOutputPort=on
  Anti-windup gain : Gain  Gain=sqrt(Ki/Kd)
  Integrator : Integrator  ExternalReset=either
  Ki : Gain  Gain=Ki
  Scope : Scope  NumInputPorts=2
  Sum5 : Sum  Inputs=-+|
  XOR : Logic  Operator=XOR  IconShape=distinctive  AllPortsSameDT=off  OutDataTypeStr=boolean
  Out1 : Outport  OutputWhenDisabled=reset  InitialOutput=0  VectorParamsAs1DForOutWhenUnconnected=off
  wires:
  eh/1 -> Ki/1
  Integrator/1 -> Out1/1
  XOR/1 -> Integrator/2
  leaderChange/1 -> XOR/1
  Enable/1 -> XOR/2
  Sum5/1 -> Integrator/1, Scope/2
  Ki/1 -> Sum5/2
  Anti-windup gain/1 -> Sum5/1, Scope/1
  inputDiff/1 -> Anti-windup gain/1

== system full_maneuver_platoon/Fd/CACC origin lane/Controller Real Leader/Veh Following/integralTerm ==
  eh : Inport
  inputDiff : Inport  Port=2
  leaderChange : Inport  Port=3
  Enable : EnablePort  ShowOutputPort=on
  Anti-windup gain : Gain  Gain=sqrt(Ki/Kd)
  Integrator : Integrator  ExternalReset=either
  Ki : Gain  Gain=Ki
  Scope : Scope  NumInputPorts=2
  Sum5 : Sum  Inputs=-+|
  XOR : Logic  Operator=XOR  IconShape=distinctive  AllPortsSameDT=off  OutDataTypeStr=boolean
  Out1 : Outport  OutputWhenDisabled=reset  InitialOutput=0  VectorParamsAs1DForOutWhenUnconnected=off
  wires:
  eh/1 -> Ki/1
  Integrator/1 -> Out1/1
  XOR/1 -> Integrator/2
  leaderChange/1 -> XOR/1
  Enable/1 -> XOR/2
  Sum5/1 -> Integrator/1, Scope/2
  Ki/1 -> Sum5/2
  Anti-windup gain/1 -> Sum5/1, Scope/1
  inputDiff/1 -> Anti-windup gain/1

== system full_maneuver_platoon/Fd/CACC origin lane/Controller Real Leader/Velocity Control/integral term ==
  ev : Inport
  integralReset : Inport  Port=2
  Enable : EnablePort  StatesWhenEnabling=reset
  Integrator2 : Integrator  ExternalReset=rising
  velKi : Gain  Gain=velKi
  Out1 : Outport  OutputWhenDisabled=reset  InitialOutput=0
  wires:
  integralReset/1 -> Integrator2/2
  velKi/1 -> Integrator2/1
  Integrator2/1 -> Out1/1
  ev/1 -> velKi/1

== system full_maneuver_platoon/Fo/CACC origin lane/Controller Real Leader/Veh Following/integralTerm ==
  eh : Inport
  inputDiff : Inport  Port=2
  leaderChange : Inport  Port=3
  Enable : EnablePort  ShowOutputPort=on
  Anti-windup gain : Gain  Gain=sqrt(Ki/Kd)
  Integrator : Integrator  ExternalReset=either
  Ki : Gain  Gain=Ki
  Scope : Scope  NumInputPorts=2
  Sum5 : Sum  Inputs=-+|
  XOR : Logic  Operator=XOR  IconShape=distinctive  AllPortsSameDT=off  OutDataTypeStr=boolean
  Out1 : Outport  OutputWhenDisabled=reset  InitialOutput=0  VectorParamsAs1DForOutWhenUnconnected=off
  wires:
  inputDiff/1 -> Anti-windup gain/1
  Anti-windup gain/1 -> Scope/1, Sum5/1
  Ki/1 -> Sum5/2
  Sum5/1 -> Scope/2, Integrator/1
  Enable/1 -> XOR/2
  leaderChange/1 -> XOR/1
  XOR/1 -> Integrator/2
  Integrator/1 -> Out1/1
  eh/1 -> Ki/1

== system full_maneuver_platoon/Fo/CACC origin lane/Controller Real Leader/Velocity Control/integral term ==
  ev : Inport
  integralReset : Inport  Port=2
  Enable : EnablePort  StatesWhenEnabling=reset
  Integrator2 : Integrator  ExternalReset=rising
  velKi : Gain  Gain=velKi
  Out1 : Outport  OutputWhenDisabled=reset  InitialOutput=0
  wires:
  ev/1 -> velKi/1
  Integrator2/1 -> Out1/1
  velKi/1 -> Integrator2/1
  integralReset/1 -> Integrator2/2

== system full_maneuver_platoon/Ld/CACC origin lane/Controller Real Leader/Veh Following/integralTerm ==
  eh : Inport
  inputDiff : Inport  Port=2
  leaderChange : Inport  Port=3
  Enable : EnablePort  ShowOutputPort=on
  Anti-windup gain : Gain  Gain=sqrt(Ki/Kd)
  Integrator : Integrator  ExternalReset=either
  Ki : Gain  Gain=Ki
  Scope : Scope  NumInputPorts=2
  Sum5 : Sum  Inputs=-+|
  XOR : Logic  Operator=XOR  IconShape=distinctive  AllPortsSameDT=off  OutDataTypeStr=boolean
  Out1 : Outport  OutputWhenDisabled=reset  InitialOutput=0  VectorParamsAs1DForOutWhenUnconnected=off
  wires:
  inputDiff/1 -> Anti-windup gain/1
  Anti-windup gain/1 -> Scope/1, Sum5/1
  Ki/1 -> Sum5/2
  Sum5/1 -> Scope/2, Integrator/1
  Enable/1 -> XOR/2
  leaderChange/1 -> XOR/1
  XOR/1 -> Integrator/2
  Integrator/1 -> Out1/1
  eh/1 -> Ki/1

== system full_maneuver_platoon/Ld/CACC origin lane/Controller Real Leader/Velocity Control/integral term ==
  ev : Inport
  integralReset : Inport  Port=2
  Enable : EnablePort  StatesWhenEnabling=reset
  Integrator2 : Integrator  ExternalReset=rising
  velKi : Gain  Gain=velKi
  Out1 : Outport  OutputWhenDisabled=reset  InitialOutput=0
  wires:
  ev/1 -> velKi/1
  Integrator2/1 -> Out1/1
  velKi/1 -> Integrator2/1
  integralReset/1 -> Integrator2/2

== system full_maneuver_platoon/Lo/CACC origin lane/Controller Real Leader/Veh Following/integralTerm ==
  eh : Inport
  inputDiff : Inport  Port=2
  leaderChange : Inport  Port=3
  Enable : EnablePort  ShowOutputPort=on
  Anti-windup gain : Gain  Gain=sqrt(Ki/Kd)
  Integrator : Integrator  ExternalReset=either
  Ki : Gain  Gain=Ki
  Scope : Scope  NumInputPorts=2
  Sum5 : Sum  Inputs=-+|
  XOR : Logic  Operator=XOR  IconShape=distinctive  AllPortsSameDT=off  OutDataTypeStr=boolean
  Out1 : Outport  OutputWhenDisabled=reset  InitialOutput=0  VectorParamsAs1DForOutWhenUnconnected=off
  wires:
  eh/1 -> Ki/1
  Integrator/1 -> Out1/1
  XOR/1 -> Integrator/2
  leaderChange/1 -> XOR/1
  Enable/1 -> XOR/2
  Sum5/1 -> Integrator/1, Scope/2
  Ki/1 -> Sum5/2
  Anti-windup gain/1 -> Sum5/1, Scope/1
  inputDiff/1 -> Anti-windup gain/1

== system full_maneuver_platoon/Lo/CACC origin lane/Controller Real Leader/Velocity Control/integral term ==
  ev : Inport
  integralReset : Inport  Port=2
  Enable : EnablePort  StatesWhenEnabling=reset
  Integrator2 : Integrator  ExternalReset=rising
  velKi : Gain  Gain=velKi
  Out1 : Outport  OutputWhenDisabled=reset  InitialOutput=0
  wires:
  integralReset/1 -> Integrator2/2
  velKi/1 -> Integrator2/1
  Integrator2/1 -> Out1/1
  ev/1 -> velKi/1

== system full_maneuver_platoon/p1/CACC destination lane/Virtual Vehicle Following/Min Velocity Control/integral term ==
  ev : Inport
  intergralReset : Inport  Port=2
  Enable : EnablePort  StatesWhenEnabling=reset
  Integrator2 : Integrator  ExternalReset=rising
  velKi : Gain  Gain=velKi
  Out1 : Outport  OutputWhenDisabled=reset  InitialOutput=0
  wires:
  ev/1 -> velKi/1
  Integrator2/1 -> Out1/1
  velKi/1 -> Integrator2/1
  intergralReset/1 -> Integrator2/2

== system full_maneuver_platoon/p1/CACC destination lane/Virtual Vehicle Following/Virtual Leader Following/integralTerm ==
  eh : Inport
  inputDiff : Inport  Port=2
  leaderChange : Inport  Port=3
  Enable : EnablePort  ShowOutputPort=on
  Anti-windup gain : Gain  Gain=sqrt(Ki/Kd)
  Integrator : Integrator  ExternalReset=either
  Ki : Gain  Gain=Ki
  Scope : Scope  NumInputPorts=2
  Sum5 : Sum  Inputs=-+|
  XOR : Logic  Operator=XOR  IconShape=distinctive  AllPortsSameDT=off  OutDataTypeStr=boolean
  Out1 : Outport  OutputWhenDisabled=reset  InitialOutput=0  VectorParamsAs1DForOutWhenUnconnected=off
  wires:
  inputDiff/1 -> Anti-windup gain/1
  Anti-windup gain/1 -> Scope/1, Sum5/1
  Ki/1 -> Sum5/2
  Sum5/1 -> Scope/2, Integrator/1
  Enable/1 -> XOR/2
  leaderChange/1 -> XOR/1
  XOR/1 -> Integrator/2
  Integrator/1 -> Out1/1
  eh/1 -> Ki/1

== system full_maneuver_platoon/p2/CACC destination lane/Virtual Vehicle Following/Min Velocity Control/integral term ==
  ev : Inport
  intergralReset : Inport  Port=2
  Enable : EnablePort  StatesWhenEnabling=reset
  Integrator2 : Integrator  ExternalReset=rising
  velKi : Gain  Gain=velKi
  Out1 : Outport  OutputWhenDisabled=reset  InitialOutput=0
  wires:
  intergralReset/1 -> Integrator2/2
  velKi/1 -> Integrator2/1
  Integrator2/1 -> Out1/1
  ev/1 -> velKi/1

== system full_maneuver_platoon/p2/CACC destination lane/Virtual Vehicle Following/Virtual Leader Following/integralTerm ==
  eh : Inport
  inputDiff : Inport  Port=2
  leaderChange : Inport  Port=3
  Enable : EnablePort  ShowOutputPort=on
  Anti-windup gain : Gain  Gain=sqrt(Ki/Kd)
  Integrator : Integrator  ExternalReset=either
  Ki : Gain  Gain=Ki
  Scope : Scope  NumInputPorts=2
  Sum5 : Sum  Inputs=-+|
  XOR : Logic  Operator=XOR  IconShape=distinctive  AllPortsSameDT=off  OutDataTypeStr=boolean
  Out1 : Outport  OutputWhenDisabled=reset  InitialOutput=0  VectorParamsAs1DForOutWhenUnconnected=off
  wires:
  eh/1 -> Ki/1
  Integrator/1 -> Out1/1
  XOR/1 -> Integrator/2
  leaderChange/1 -> XOR/1
  Enable/1 -> XOR/2
  Sum5/1 -> Integrator/1, Scope/2
  Ki/1 -> Sum5/2
  Anti-windup gain/1 -> Sum5/1, Scope/1
  inputDiff/1 -> Anti-windup gain/1

== system full_maneuver_platoon/p3/CACC destination lane/Virtual Vehicle Following/Min Velocity Control/integral term ==
  ev : Inport
  intergralReset : Inport  Port=2
  Enable : EnablePort  StatesWhenEnabling=reset
  Integrator2 : Integrator  ExternalReset=rising
  velKi : Gain  Gain=velKi
  Out1 : Outport  OutputWhenDisabled=reset  InitialOutput=0
  wires:
  ev/1 -> velKi/1
  Integrator2/1 -> Out1/1
  velKi/1 -> Integrator2/1
  intergralReset/1 -> Integrator2/2

== system full_maneuver_platoon/p3/CACC destination lane/Virtual Vehicle Following/Virtual Leader Following/integralTerm ==
  eh : Inport
  inputDiff : Inport  Port=2
  leaderChange : Inport  Port=3
  Enable : EnablePort  ShowOutputPort=on
  Anti-windup gain : Gain  Gain=sqrt(Ki/Kd)
  Integrator : Integrator  ExternalReset=either
  Ki : Gain  Gain=Ki
  Scope : Scope  NumInputPorts=2
  Sum5 : Sum  Inputs=-+|
  XOR : Logic  Operator=XOR  IconShape=distinctive  AllPortsSameDT=off  OutDataTypeStr=boolean
  Out1 : Outport  OutputWhenDisabled=reset  InitialOutput=0  VectorParamsAs1DForOutWhenUnconnected=off
  wires:
  inputDiff/1 -> Anti-windup gain/1
  Anti-windup gain/1 -> Scope/1, Sum5/1
  Ki/1 -> Sum5/2
  Sum5/1 -> Scope/2, Integrator/1
  Enable/1 -> XOR/2
  leaderChange/1 -> XOR/1
  XOR/1 -> Integrator/2
  Integrator/1 -> Out1/1
  eh/1 -> Ki/1
